simulink subsystem "GemeloDigitalZ"  (R2023b)
settings: Solver=VariableStepAuto  StartTime=0.0  StopTime=10.0  RelTol=1e-3
settings Model: Creator=Carlos  LastModifiedBy=Carlos

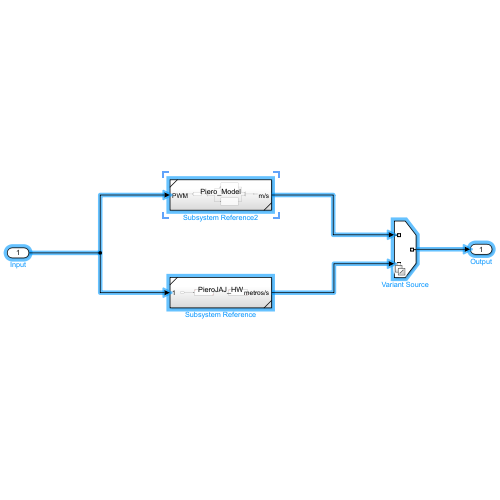
[thumbnail: Simulink's stored preview of the top-level diagram]
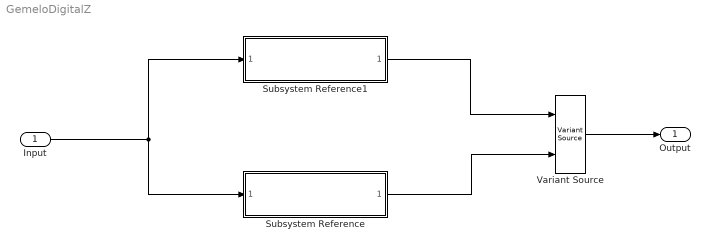
== system GemeloDigitalZ ==
  Input : Inport
  Subsystem Reference : Subsystem  ReferencedSubsystem=PieroJAJ_HW
  Subsystem Reference1 : Subsystem  ReferencedSubsystem=Piero_ModelZ
  Variant Source : VariantSource  VariantControlMode=sim codegen switching
  Output : Outport
  wires:
  Variant Source/1 -> Output/1
  Subsystem Reference1/1 -> Variant Source/1
  Subsystem Reference/1 -> Variant Source/2
  Input/1 -> Subsystem Reference/1, Subsystem Reference1/1
